simulink model "Sim_LabVaja1_6"  (R2019b)
settings: Solver=VariableStepAuto  StartTime=0.0  StopTime=1600  RelTol=1e-3
values from neighbouring files (symbols this model uses):
  kv1 = 0.1    [LaboratorijskaVaja1_6.m]    (also in odvod.m)
  kv2 = 0.05    [LaboratorijskaVaja1_6.m]    (also in odvod.m)
  ro = 1000    [LaboratorijskaVaja1_1.m]    (also in LaboratorijskaVaja1_2_3.m; LaboratorijskaVaja1_4.m; LaboratorijskaVaja1_6.m; odvod.m)
  S1 = 0.01    [LaboratorijskaVaja1_1.m]    (also in LaboratorijskaVaja1_2_3.m; LaboratorijskaVaja1_4.m; LaboratorijskaVaja1_6.m; odvod.m)
  S2 = 0.01    [LaboratorijskaVaja1_1.m]    (also in LaboratorijskaVaja1_2_3.m; LaboratorijskaVaja1_4.m; LaboratorijskaVaja1_6.m; odvod.m)
undefined symbols (not defined in the file or in its folder): sgn
settings Model: Creator=bonce  LastModifiedBy=bonce
settings DataIOCC: ReturnWorkspaceOutputs=off

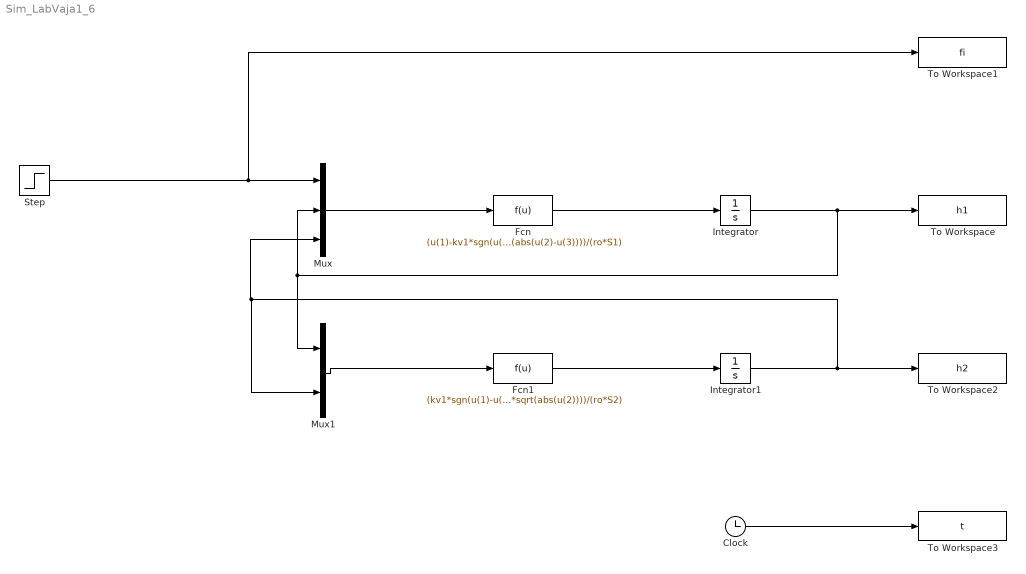
== system Sim_LabVaja1_6 ==
  Clock : Clock
  Fcn : Fcn  Expr=(u(1)-kv1*sgn(u(2) - u(3))*sqrt(abs(u(2)-u(3))))/(ro*S1)
  Fcn1 : Fcn  Expr=(kv1*sgn(u(1)-u(2))*sqrt(abs((u(1)-u(2))))-kv2*sgn(u(2))*sqrt(abs(u(2))))/(ro*S2)
  Integrator : Integrator
  Integrator1 : Integrator
  Mux : Mux  Inputs=3
  Mux1 : Mux  Inputs=2
  Step : Step  Time=0  After=0.02  SampleTime=1600
  To Workspace : ToWorkspace  VariableName=h1  SampleTime=-1
  To Workspace1 : ToWorkspace  VariableName=fi  SampleTime=-1
  To Workspace2 : ToWorkspace  VariableName=h2  SampleTime=-1
  To Workspace3 : ToWorkspace  VariableName=t  SampleTime=-1
  wires:
  Step/1 -> To Workspace1/1, Mux/1
  Mux/1 -> Fcn/1
  Fcn/1 -> Integrator/1
  Clock/1 -> To Workspace3/1
  Fcn1/1 -> Integrator1/1
  Mux1/1 -> Fcn1/1
  Integrator/1 -> Mux/2, Mux1/1, To Workspace/1
  Integrator1/1 -> Mux1/2, Mux/3, To Workspace2/1
